simulink model "process"  (R2023b)
settings: Solver=VariableStepAuto  StartTime=0.0  StopTime=inf  RelTol=1e-3
libraries: ros2lib x4
settings Model: Creator=basten  LastModifiedBy=basten

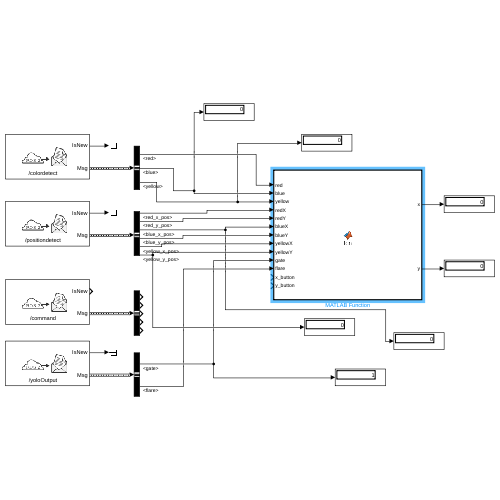
[thumbnail: Simulink's stored preview of the top-level diagram]
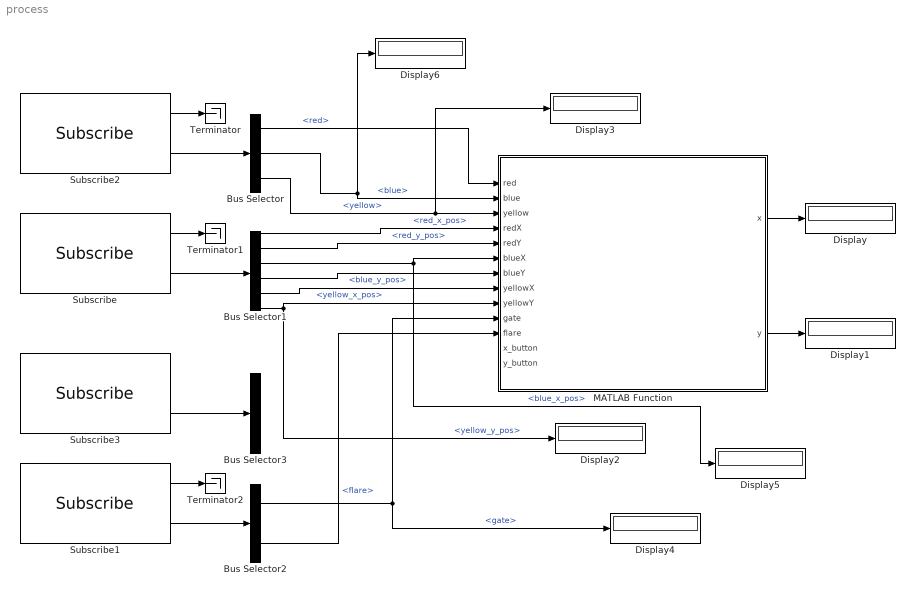
== system process ==
  Bus Selector : BusSelector  OutputSignals=red,blue,yellow
  Bus Selector1 : BusSelector  OutputSignals=red_x_pos,red_y_pos,blue_x_pos,blue_y_pos,yellow_x_pos,yellow_y_pos
  Bus Selector2 : BusSelector  OutputSignals=gate,flare
  Bus Selector3 : BusSelector  OutputSignals=x_cmd,y_cmd,yaw,depth,x_button
  Display{,1..6} (7 alike) : Display
  MATLAB Function : MATLAB Function  TreatAsAtomicUnit=on
  Subscribe : ros2lib/Subscribe  topicSource=Specify your own  topic=/positiondetect  messageType=tugas_opencv/Position  sampleTime=0.01  QOSHistory=Keep last  QOSDepth=1  QOSReliability=Reliable  QOSDurability=Volatile
  Subscribe1 : ros2lib/Subscribe  topicSource=Specify your own  topic=/yoloOutput  messageType=tugas_yolo_yolocpp/Seen  sampleTime=0.01  QOSHistory=Keep last  QOSDepth=1  QOSReliability=Reliable  QOSDurability=Volatile
  Subscribe2 : ros2lib/Subscribe  topicSource=Specify your own  topic=/colordetect  messageType=tugas_opencv/Color  sampleTime=0.01  QOSHistory=Keep last  QOSDepth=1  QOSReliability=Reliable  QOSDurability=Volatile
  Subscribe3 : ros2lib/Subscribe  topicSource=Specify your own  topic=/command  messageType=tugas_joy/Command  sampleTime=0.01  QOSHistory=Keep last  QOSDepth=1  QOSReliability=Reliable  QOSDurability=Volatile
  Terminator : Terminator
  Terminator1 : Terminator
  Terminator2 : Terminator
  wires:
  Subscribe2/2 -> Bus Selector/1
  Subscribe/2 -> Bus Selector1/1
  Subscribe1/2 -> Bus Selector2/1
  Bus Selector/1 -> MATLAB Function/1(red)  "<red>"
  Bus Selector/2 -> Display6/1, MATLAB Function/2(blue)  "<blue>"
  Bus Selector/3 -> Display3/1, MATLAB Function/3(yellow)  "<yellow>"
  Bus Selector1/1 -> MATLAB Function/4(redX)  "<red_x_pos>"
  Bus Selector1/2 -> MATLAB Function/5(redY)  "<red_y_pos>"
  Bus Selector1/3 -> Display5/1, MATLAB Function/6(blueX)  "<blue_x_pos>"
  Bus Selector1/4 -> MATLAB Function/7(blueY)  "<blue_y_pos>"
  Bus Selector1/5 -> MATLAB Function/8(yellowX)  "<yellow_x_pos>"
  Bus Selector1/6 -> Display2/1, MATLAB Function/9(yellowY)  "<yellow_y_pos>"
  Bus Selector2/1 -> MATLAB Function/10(gate), Display4/1  "<gate>"
  Bus Selector2/2 -> MATLAB Function/11(flare)  "<flare>"
  MATLAB Function/1(x) -> Display/1
  MATLAB Function/2(y) -> Display1/1
  Subscribe1/1 -> Terminator2/1
  Subscribe/1 -> Terminator1/1
  Subscribe2/1 -> Terminator/1
  Subscribe3/2 -> Bus Selector3/1

== matlab function process/MATLAB Function ==
  data: x output; red input; y output; blue input; yellow input; redX input; redY input; blueX input; blueY input; yellowX input; yellowY input; gate input; flare input; x_button input; y_button input
function [x, y] = fcn(red, blue, yellow, redX, redY, blueX, blueY, yellowX, yellowY, gate, flare, x_button, y_button)

x = int32(0);
y = int32(0);



persistent currentColor;

if isempty(currentColor)
    currentColor = colorEnum.RED;
end

enumList = enumeration('colorEnum');
currentIndex = find(enumList == currentColor);
currentIndex = currentIndex(1);

nextIndex = mod(currentIndex,3) + 1;

disp(x);
    
if y_button == 1
    

    if currentColor == enumList(currentIndex) && red
        
        while (redX <-20) || (redX > 20)

            if redX < 0
                x = int32(-100);
            end
            if redX > 0
                x = int32(100);
            end
        end
        currentColor = enumList(nextIndex);
    
    end
    
    if currentColor == enumList(nextIndex) && yellow
        
        while yellowX <-20 || yellowX > 20
            if yellowX < 0
                x = int32(-100);
            end
            if yellowX > 0
                x = int32(100);
            end
        end
        currentColor = enumList(nextIndex + 1);
    
    end
    
    if currentColor == enumList(nextIndex + 1) && blue
        
        while blueX <-20 || blueX > 20
            if blueX < 0
                x = int32(-100);
            end
            if blueX > 0
                x = int32(100);
            end
        end
        currentColor = colorEnum.RED;
    
    end
end
